simulink model "Q7_cartesian_space_solution"  (R2017a)
settings: Solver=FixedStepAuto  StartTime=0.0  StopTime=10  FixedStep=0.001  RelTol=0.00001
model workspace (MAT data in the model file):
  a_1 = 1
  a_2 = 1
  g = 9.8
  m_1 = 1
  m_2 = 1
  simulation_time = 4
  x1_0 = 1.9998
  x1_dot_0 = 0
  x1_dot_f = 0
  x1_double_dot_0 = 0
  x1_double_dot_f = 0
  x1_f = 0
  x2_0 = 0
  x2_dot_0 = 0
  x2_dot_f = 0
  x2_double_dot_0 = 0
  x2_double_dot_f = 0
  x2_f = 1
libraries: simulink x15
settings Model: Creator=Omer  LastModifiedBy=Omer
settings ModelReferenceCC: ModelReferenceMinAlgLoopOccurrences=on

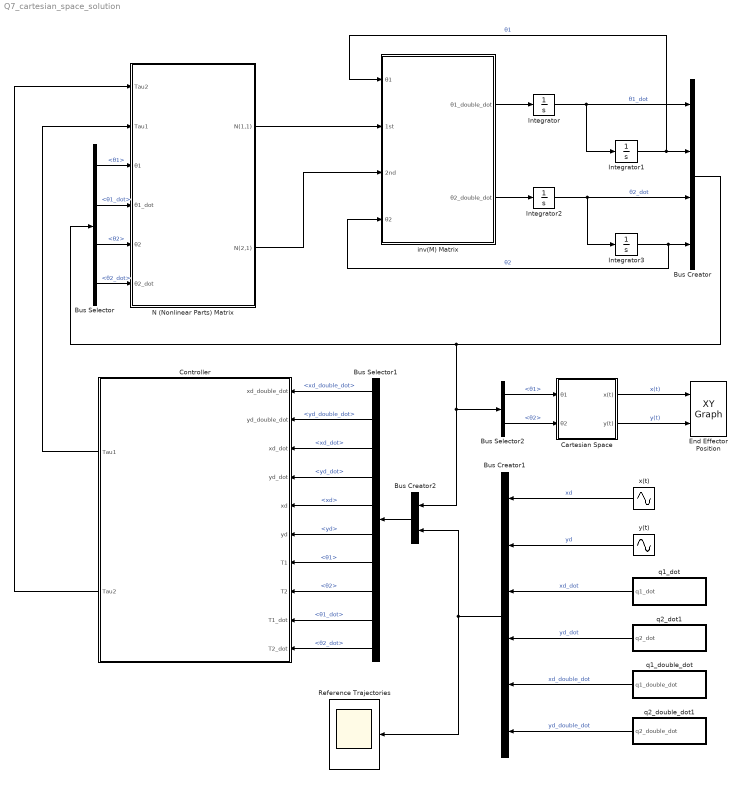
== system Q7_cartesian_space_solution ==
  Bus Creator : BusCreator  Inputs=4
  Bus Creator1 : BusCreator  Inputs=6
  Bus Creator2 : BusCreator  Inputs=2
  Bus Selector : BusSelector  OutputSignals=θ1,θ1_dot,θ2,θ2_dot
  Bus Selector1 : BusSelector  OutputSignals=signal2.xd_double_dot,signal2.yd_double_dot,signal2.xd_dot,signal2.yd_dot,signal2.xd,signal2.yd,signal1.θ1,signal1.θ2,signal1.θ1_dot,signal1.θ2_dot
  Bus Selector2 : BusSelector  OutputSignals=θ1,θ2
  "Cartesian Space " : Subsystem  TreatAsAtomicUnit=on
  Controller : MATLAB Function  TreatAsAtomicUnit=on
  End Effector Position : simulink/Sinks/XY Graph  xmin=-2  xmax=2  ymin=-1  ymax=2  st=-1
  Integrator : Integrator  UpperSaturationLimit=5  LowerSaturationLimit=-5
  Integrator1 : Integrator  InitialCondition=pi/6  UpperSaturationLimit=5  LowerSaturationLimit=-5
  Integrator2 : Integrator  UpperSaturationLimit=5  LowerSaturationLimit=-5
  Integrator3 : Integrator  InitialCondition=5*pi/6  UpperSaturationLimit=5  LowerSaturationLimit=-5
  N (Nonlinear Parts) Matrix : Subsystem  TreatAsAtomicUnit=on
  Reference Trajectories : Scope
  inv(M) Matrix : Subsystem  TreatAsAtomicUnit=on
  q1_dot : Subsystem  TreatAsAtomicUnit=on
  q1_double_dot : Subsystem  TreatAsAtomicUnit=on
  q2_dot1 : Subsystem  TreatAsAtomicUnit=on
  q2_double_dot1 : Subsystem  TreatAsAtomicUnit=on
  x(t) : Sin  Amplitude=0.5  Frequency=pi/5  SampleTime=0
  y(t) : Sin  Amplitude=0.5  Bias=1  Frequency=pi/5  Phase=-pi/2  SampleTime=0
  wires:
  N (Nonlinear Parts) Matrix/2(N(2,1)) -> inv(M) Matrix/3(2nd)
  N (Nonlinear Parts) Matrix/1(N(1,1)) -> inv(M) Matrix/2(1st)
  Bus Creator/1 -> Bus Selector2/1, Bus Creator2/1, Bus Selector/1
  inv(M) Matrix/2(θ2_double_dot) -> Integrator2/1
  Bus Selector/1 -> N (Nonlinear Parts) Matrix/3("θ1 ")  "<θ1>"
  Integrator2/1 -> Integrator3/1, Bus Creator/3  "θ2_dot"
  Integrator3/1 -> inv(M) Matrix/4(θ2), Bus Creator/4  "θ2"
  Integrator1/1 -> inv(M) Matrix/1(θ1), Bus Creator/2  "θ1"
  Bus Selector/3 -> N (Nonlinear Parts) Matrix/5(θ2)  "<θ2>"
  Bus Selector/2 -> N (Nonlinear Parts) Matrix/4(θ1_dot)  "<θ1_dot>"
  Integrator/1 -> Bus Creator/1, Integrator1/1  "θ1_dot"
  Bus Selector/4 -> N (Nonlinear Parts) Matrix/6(θ2_dot)  "<θ2_dot>"
  inv(M) Matrix/1(θ1_double_dot) -> Integrator/1
  Bus Selector2/1 -> "Cartesian Space "/1(θ1)  "<θ1>"
  Bus Selector2/2 -> "Cartesian Space "/2(θ2)  "<θ2>"
  "Cartesian Space "/1(x(t)) -> End Effector Position/1  "x(t)"
  "Cartesian Space "/2(y(t)) -> End Effector Position/2  "y(t)"
  Bus Creator2/1 -> Bus Selector1/1
  Bus Selector1/1 -> Controller/1(xd_double_dot)  "<xd_double_dot>"
  Bus Selector1/2 -> Controller/2(yd_double_dot)  "<yd_double_dot>"
  Bus Selector1/3 -> Controller/3(xd_dot)  "<xd_dot>"
  Bus Selector1/4 -> Controller/4(yd_dot)  "<yd_dot>"
  Bus Selector1/5 -> Controller/5(xd)  "<xd>"
  Bus Selector1/6 -> Controller/6(yd)  "<yd>"
  Bus Selector1/7 -> Controller/7(T1)  "<θ1>"
  Bus Selector1/8 -> Controller/8(T2)  "<θ2>"
  Bus Selector1/9 -> Controller/9(T1_dot)  "<θ1_dot>"
  Bus Selector1/10 -> Controller/10(T2_dot)  "<θ2_dot>"
  Controller/1(Tau1) -> N (Nonlinear Parts) Matrix/2(Tau1)
  Controller/2(Tau2) -> N (Nonlinear Parts) Matrix/1(Tau2)
  x(t)/1 -> Bus Creator1/1  "xd"
  q1_double_dot/1(q1_double_dot) -> Bus Creator1/5  "xd_double_dot"
  q2_dot1/1(q2_dot) -> Bus Creator1/4  "yd_dot"
  Bus Creator1/1 -> Reference Trajectories/1, Bus Creator2/2
  q2_double_dot1/1(q2_double_dot) -> Bus Creator1/6  "yd_double_dot"
  y(t)/1 -> Bus Creator1/2  "yd"
  q1_dot/1(q1_dot) -> Bus Creator1/3  "xd_dot"

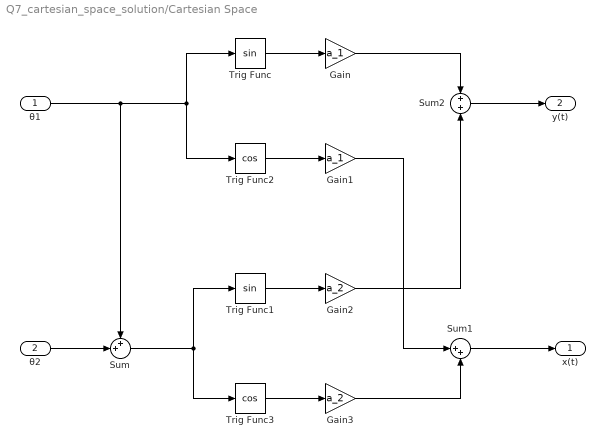
== system Q7_cartesian_space_solution/Cartesian Space  ==
  θ1 : Inport
  θ2 : Inport  Port=2
  Gain : Gain  Gain=a_1
  Gain1 : Gain  Gain=a_1
  Gain2 : Gain  Gain=a_2
  Gain3 : Gain  Gain=a_2
  Sum : Sum  Inputs=++|
  Sum1 : Sum  Inputs=|++
  Sum2 : Sum  Inputs=+|+
  Trig Func : Trigonometry
  Trig Func1 : Trigonometry
  Trig Func2 : Trigonometry  Operator=cos
  Trig Func3 : Trigonometry  Operator=cos
  x(t) : Outport
  y(t) : Outport  Port=2
  wires:
  θ1/1 -> Trig Func2/1, Trig Func/1, Sum/1
  θ2/1 -> Sum/2
  Sum/1 -> Trig Func3/1, Trig Func1/1
  Sum2/1 -> y(t)/1
  Sum1/1 -> x(t)/1
  Trig Func/1 -> Gain/1
  Gain/1 -> Sum2/1
  Trig Func2/1 -> Gain1/1
  Gain1/1 -> Sum1/1
  Trig Func1/1 -> Gain2/1
  Gain2/1 -> Sum2/2
  Trig Func3/1 -> Gain3/1
  Gain3/1 -> Sum1/2

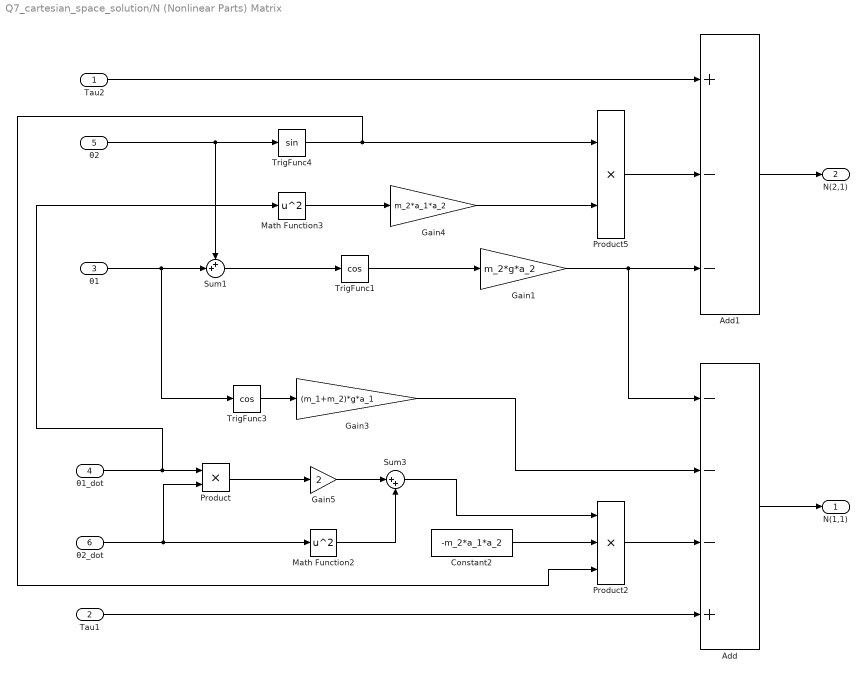
== system Q7_cartesian_space_solution/N (Nonlinear Parts) Matrix ==
  Tau2 : Inport
  Tau1 : Inport  Port=2
  "θ1 " : Inport  Port=3
  θ1_dot : Inport  Port=4
  θ2 : Inport  Port=5
  θ2_dot : Inport  Port=6
  Add : Sum  Inputs=---+
  Add1 : Sum  Inputs=+--
  Constant2 : Constant  Value=-m_2*a_1*a_2
  Gain1 : Gain  Gain=m_2*g*a_2
  Gain3 : Gain  Gain=(m_1+m_2)*g*a_1
  Gain4 : Gain  Gain=m_2*a_1*a_2
  Gain5 : Gain  Gain=2
  Math Function2 : Math  Operator=square  SaturateOnIntegerOverflow=on
  Math Function3 : Math  Operator=square  SaturateOnIntegerOverflow=on
  Product : Product
  Product2 : Product  Inputs=3
  Product5 : Product
  Sum1 : Sum  Inputs=++|
  Sum3 : Sum  Inputs=|++
  TrigFunc1 : Trigonometry  Operator=cos
  TrigFunc3 : Trigonometry  Operator=cos
  TrigFunc4 : Trigonometry
  N(1,1) : Outport
  N(2,1) : Outport  Port=2
  wires:
  Product2/1 -> Add/3
  Gain3/1 -> Add/2
  θ2/1 -> TrigFunc4/1, Sum1/1
  TrigFunc4/1 -> Product2/3, Product5/1
  Add1/1 -> N(2,1)/1
  Math Function3/1 -> Gain4/1
  θ1_dot/1 -> Product/1, Math Function3/1
  θ2_dot/1 -> Product/2, Math Function2/1
  Sum1/1 -> TrigFunc1/1
  Add/1 -> N(1,1)/1
  Sum3/1 -> Product2/1
  Math Function2/1 -> Sum3/2
  Tau2/1 -> Add1/1
  Constant2/1 -> Product2/2
  TrigFunc3/1 -> Gain3/1
  TrigFunc1/1 -> Gain1/1
  "θ1 "/1 -> TrigFunc3/1, Sum1/2
  Product5/1 -> Add1/2
  Tau1/1 -> Add/4
  Gain4/1 -> Product5/2
  Gain1/1 -> Add1/3, Add/1
  Product/1 -> Gain5/1
  Gain5/1 -> Sum3/1

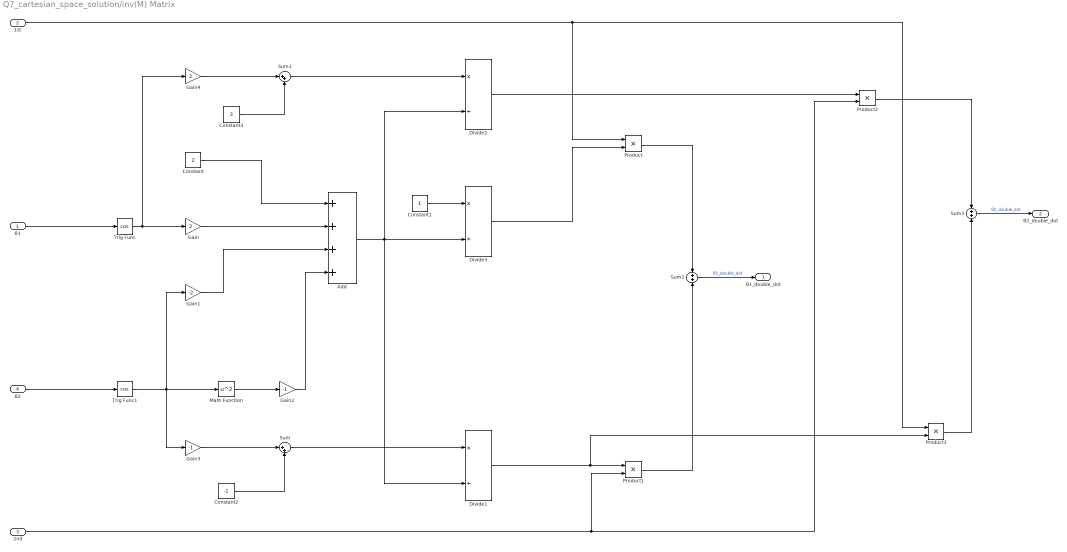
== system Q7_cartesian_space_solution/inv(M) Matrix ==
  θ1 : Inport
  1st : Inport  Port=2
  2nd : Inport  Port=3
  θ2 : Inport  Port=4
  Add : Sum  Inputs=4
  Constant : Constant  Value=2
  Constant1 : Constant
  Constant2 : Constant  Value=-1
  Constant3 : Constant  Value=3
  Divide1 : Product  Inputs=*/
  Divide2 : Product  Inputs=*/
  Divide3 : Product  Inputs=*/
  Gain : Gain  Gain=2
  Gain1 : Gain  Gain=-2
  Gain2 : Gain  Gain=-1
  Gain3 : Gain  Gain=-1
  Gain4 : Gain  Gain=2
  Math Function : Math  Operator=square  SaturateOnIntegerOverflow=on
  Product{,1..3} (4 alike) : Product
  Sum : Sum  Inputs=|++
  Sum1 : Sum  Inputs=|++
  Sum2 : Sum  Inputs=+|+
  Sum3 : Sum  Inputs=+|+
  Trig Func : Trigonometry  Operator=cos
  Trig Func1 : Trigonometry  Operator=cos
  θ1_double_dot : Outport
  θ2_double_dot : Outport  Port=2
  wires:
  Add/1 -> Divide2/2, Divide3/2, Divide1/2
  θ1/1 -> Trig Func/1
  θ2/1 -> Trig Func1/1
  Trig Func1/1 -> Gain3/1, Gain1/1, Math Function/1
  Trig Func/1 -> Gain4/1, Gain/1
  Constant/1 -> Add/1
  Gain/1 -> Add/2
  Gain1/1 -> Add/3
  Constant1/1 -> Divide3/1
  Math Function/1 -> Gain2/1
  Gain2/1 -> Add/4
  Gain3/1 -> Sum/1
  Constant2/1 -> Sum/2
  Sum/1 -> Divide1/1
  Constant3/1 -> Sum1/2
  Gain4/1 -> Sum1/1
  1st/1 -> Product/1, Product3/1
  Divide3/1 -> Product/2
  Divide1/1 -> Product3/2, Product1/1
  2nd/1 -> Product2/2, Product1/2
  Product/1 -> Sum2/1
  Product1/1 -> Sum2/2
  Sum2/1 -> θ1_double_dot/1  "θ1_double_dot"
  Sum1/1 -> Divide2/1
  Divide2/1 -> Product2/1
  Product2/1 -> Sum3/1
  Sum3/1 -> θ2_double_dot/1  "θ2_double_dot"
  Product3/1 -> Sum3/2

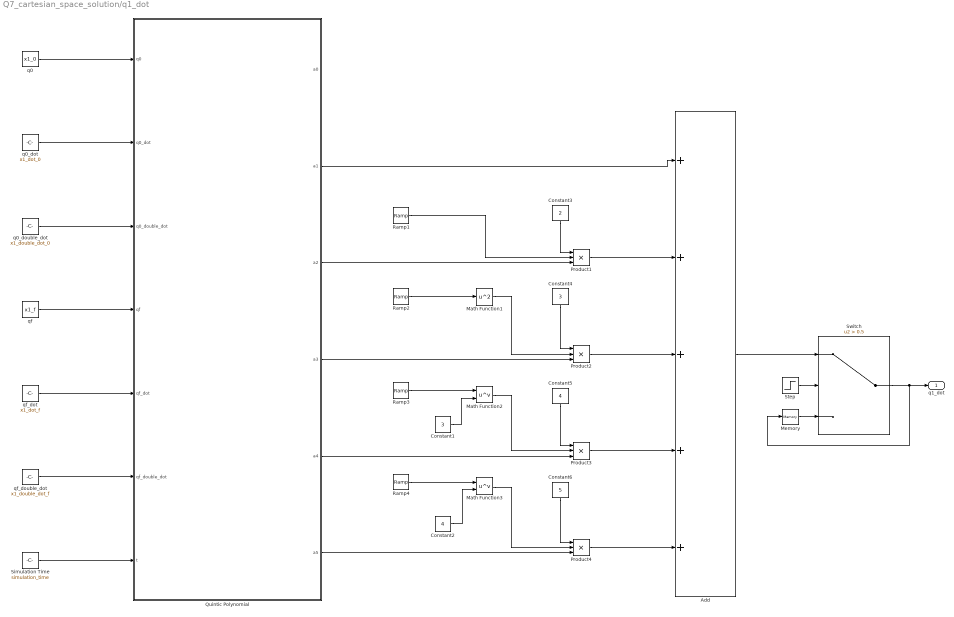
== system Q7_cartesian_space_solution/q1_dot ==
  Add : Sum  Inputs=5
  Constant1 : Constant  Value=3
  Constant2 : Constant  Value=4
  Constant3 : Constant  Value=2
  Constant4 : Constant  Value=3
  Constant5 : Constant  Value=4
  Constant6 : Constant  Value=5
  Math Function1 : Math  Operator=square  SaturateOnIntegerOverflow=on
  Math Function2 : Math  Operator=pow  SaturateOnIntegerOverflow=on
  Math Function3 : Math  Operator=pow  SaturateOnIntegerOverflow=on
  Memory : Memory
  Product{1..4} (4 alike) : Product  Inputs=3
  Quintic Polynomial : MATLAB Function  TreatAsAtomicUnit=on
  Ramp{1..4} (4 alike) : simulink/Sources/Ramp  slope=1  start=0  X0=0
  Simulation Time : Constant  Value=simulation_time
  Step : Step  Time=simulation_time  Before=1  After=0  SampleTime=0
  Switch : Switch  Criteria=u2 > Threshold  Threshold=0.5
  q0 : Constant  Value=x1_0
  q0_dot : Constant  Value=x1_dot_0
  q0_double_dot : Constant  Value=x1_double_dot_0
  qf : Constant  Value=x1_f
  qf_dot : Constant  Value=x1_dot_f
  qf_double_dot : Constant  Value=x1_double_dot_f
  q1_dot : Outport
  wires:
  Constant6/1 -> Product4/1
  Ramp1/1 -> Product1/2
  Ramp3/1 -> Math Function2/1
  Product1/1 -> Add/2
  Math Function1/1 -> Product2/2
  Simulation Time/1 -> Quintic Polynomial/7(t)
  Ramp4/1 -> Math Function3/1
  qf_double_dot/1 -> Quintic Polynomial/6(qf_double_dot)
  Quintic Polynomial/6(a5) -> Product4/3
  q0_double_dot/1 -> Quintic Polynomial/3(q0_double_dot)
  Product2/1 -> Add/3
  Quintic Polynomial/4(a3) -> Product2/3
  q0_dot/1 -> Quintic Polynomial/2(q0_dot)
  q0/1 -> Quintic Polynomial/1(q0)
  Quintic Polynomial/2(a1) -> Add/1
  Ramp2/1 -> Math Function1/1
  Math Function2/1 -> Product3/2
  Constant5/1 -> Product3/1
  Constant4/1 -> Product2/1
  Product3/1 -> Add/4
  Math Function3/1 -> Product4/2
  qf_dot/1 -> Quintic Polynomial/5(qf_dot)
  Constant3/1 -> Product1/1
  Constant1/1 -> Math Function2/2
  Constant2/1 -> Math Function3/2
  Product4/1 -> Add/5
  Quintic Polynomial/5(a4) -> Product3/3
  qf/1 -> Quintic Polynomial/4(qf)
  Quintic Polynomial/3(a2) -> Product1/3
  Memory/1 -> Switch/3
  Add/1 -> Switch/1
  Switch/1 -> q1_dot/1, Memory/1
  Step/1 -> Switch/2

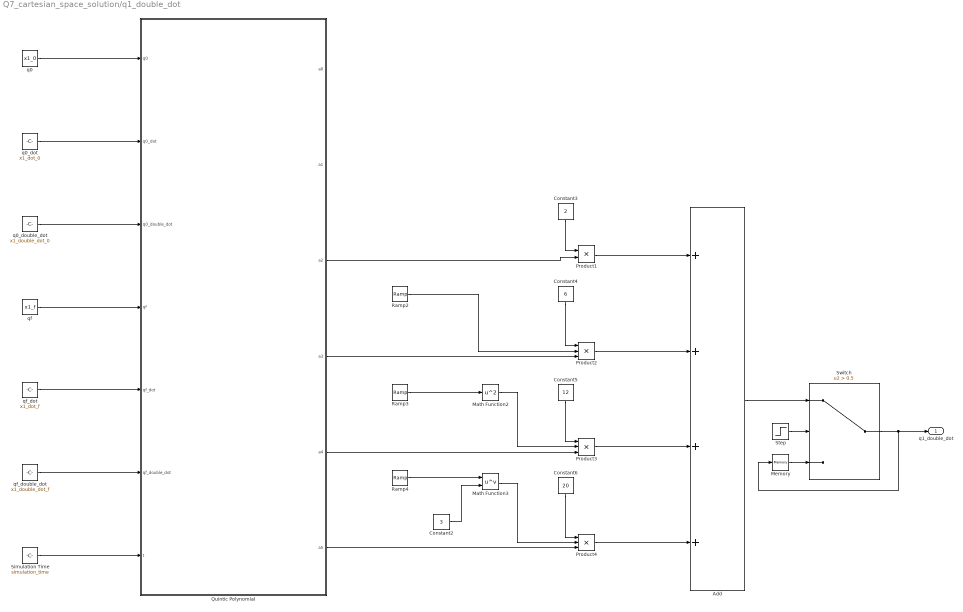
== system Q7_cartesian_space_solution/q1_double_dot ==
  Add : Sum  Inputs=4
  Constant2 : Constant  Value=3
  Constant3 : Constant  Value=2
  Constant4 : Constant  Value=6
  Constant5 : Constant  Value=12
  Constant6 : Constant  Value=20
  Math Function2 : Math  Operator=square  SaturateOnIntegerOverflow=on
  Math Function3 : Math  Operator=pow  SaturateOnIntegerOverflow=on
  Memory : Memory
  Product1 : Product
  Product2 : Product  Inputs=3
  Product3 : Product  Inputs=3
  Product4 : Product  Inputs=3
  Quintic Polynomial : MATLAB Function  TreatAsAtomicUnit=on
  Ramp2 : simulink/Sources/Ramp  slope=1  start=0  X0=0
  Ramp3 : simulink/Sources/Ramp  slope=1  start=0  X0=0
  Ramp4 : simulink/Sources/Ramp  slope=1  start=0  X0=0
  Simulation Time : Constant  Value=simulation_time
  Step : Step  Time=simulation_time  Before=1  After=0  SampleTime=0
  Switch : Switch  Criteria=u2 > Threshold  Threshold=0.5
  q0 : Constant  Value=x1_0
  q0_dot : Constant  Value=x1_dot_0
  q0_double_dot : Constant  Value=x1_double_dot_0
  qf : Constant  Value=x1_f
  qf_dot : Constant  Value=x1_dot_f
  qf_double_dot : Constant  Value=x1_double_dot_f
  q1_double_dot : Outport
  wires:
  Quintic Polynomial/6(a5) -> Product4/3
  Quintic Polynomial/5(a4) -> Product3/3
  Quintic Polynomial/4(a3) -> Product2/3
  Quintic Polynomial/3(a2) -> Product1/2
  q0_dot/1 -> Quintic Polynomial/2(q0_dot)
  Constant4/1 -> Product2/1
  Constant5/1 -> Product3/1
  Constant6/1 -> Product4/1
  Math Function3/1 -> Product4/2
  Product1/1 -> Add/1
  Constant3/1 -> Product1/1
  Math Function2/1 -> Product3/2
  Product2/1 -> Add/2
  Ramp2/1 -> Product2/2
  Ramp4/1 -> Math Function3/1
  Product3/1 -> Add/3
  qf/1 -> Quintic Polynomial/4(qf)
  qf_dot/1 -> Quintic Polynomial/5(qf_dot)
  Product4/1 -> Add/4
  q0/1 -> Quintic Polynomial/1(q0)
  Constant2/1 -> Math Function3/2
  q0_double_dot/1 -> Quintic Polynomial/3(q0_double_dot)
  Ramp3/1 -> Math Function2/1
  qf_double_dot/1 -> Quintic Polynomial/6(qf_double_dot)
  Simulation Time/1 -> Quintic Polynomial/7(t)
  Memory/1 -> Switch/3
  Add/1 -> Switch/1
  Switch/1 -> q1_double_dot/1, Memory/1
  Step/1 -> Switch/2

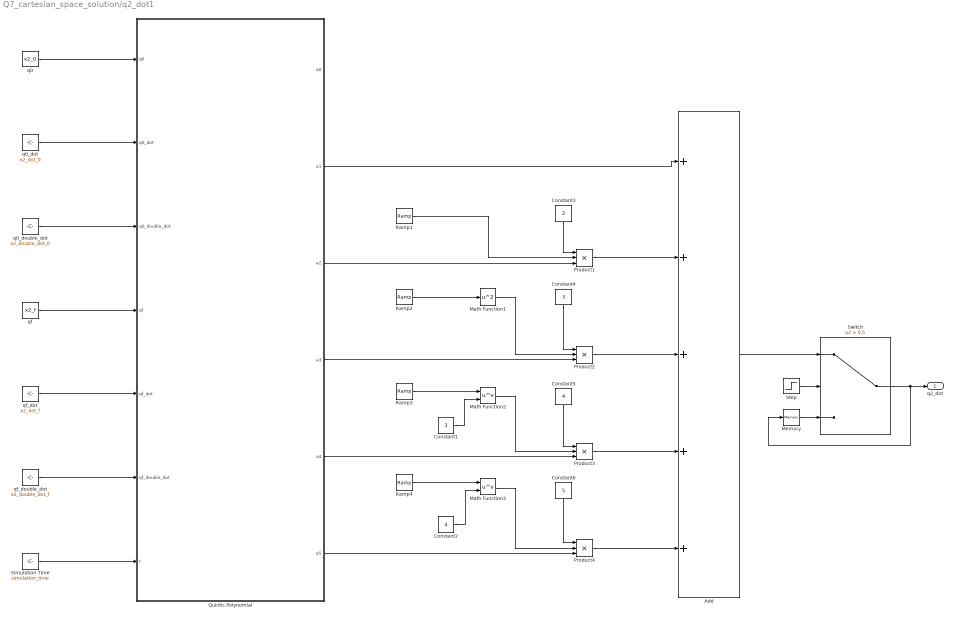
== system Q7_cartesian_space_solution/q2_dot1 ==
  Add : Sum  Inputs=5
  Constant1 : Constant  Value=3
  Constant2 : Constant  Value=4
  Constant3 : Constant  Value=2
  Constant4 : Constant  Value=3
  Constant5 : Constant  Value=4
  Constant6 : Constant  Value=5
  Math Function1 : Math  Operator=square  SaturateOnIntegerOverflow=on
  Math Function2 : Math  Operator=pow  SaturateOnIntegerOverflow=on
  Math Function3 : Math  Operator=pow  SaturateOnIntegerOverflow=on
  Memory : Memory
  Product{1..4} (4 alike) : Product  Inputs=3
  Quintic Polynomial : MATLAB Function  TreatAsAtomicUnit=on
  Ramp{1..4} (4 alike) : simulink/Sources/Ramp  slope=1  start=0  X0=0
  Simulation Time : Constant  Value=simulation_time
  Step : Step  Time=simulation_time  Before=1  After=0  SampleTime=0
  Switch : Switch  Criteria=u2 > Threshold  Threshold=0.5
  q0 : Constant  Value=x2_0
  q0_dot : Constant  Value=x2_dot_0
  q0_double_dot : Constant  Value=x2_double_dot_0
  qf : Constant  Value=x2_f
  qf_dot : Constant  Value=x2_dot_f
  qf_double_dot : Constant  Value=x2_double_dot_f
  q2_dot : Outport
  wires:
  Quintic Polynomial/2(a1) -> Add/1
  Product1/1 -> Add/2
  Product2/1 -> Add/3
  Product3/1 -> Add/4
  Product4/1 -> Add/5
  Ramp1/1 -> Product1/2
  Ramp2/1 -> Math Function1/1
  Ramp3/1 -> Math Function2/1
  Ramp4/1 -> Math Function3/1
  Quintic Polynomial/3(a2) -> Product1/3
  Math Function1/1 -> Product2/2
  Math Function2/1 -> Product3/2
  Math Function3/1 -> Product4/2
  Quintic Polynomial/4(a3) -> Product2/3
  Quintic Polynomial/5(a4) -> Product3/3
  Quintic Polynomial/6(a5) -> Product4/3
  Constant1/1 -> Math Function2/2
  Constant2/1 -> Math Function3/2
  q0/1 -> Quintic Polynomial/1(q0)
  q0_dot/1 -> Quintic Polynomial/2(q0_dot)
  q0_double_dot/1 -> Quintic Polynomial/3(q0_double_dot)
  qf/1 -> Quintic Polynomial/4(qf)
  qf_dot/1 -> Quintic Polynomial/5(qf_dot)
  qf_double_dot/1 -> Quintic Polynomial/6(qf_double_dot)
  Simulation Time/1 -> Quintic Polynomial/7(t)
  Constant3/1 -> Product1/1
  Constant4/1 -> Product2/1
  Constant5/1 -> Product3/1
  Constant6/1 -> Product4/1
  Memory/1 -> Switch/3
  Add/1 -> Switch/1
  Switch/1 -> q2_dot/1, Memory/1
  Step/1 -> Switch/2

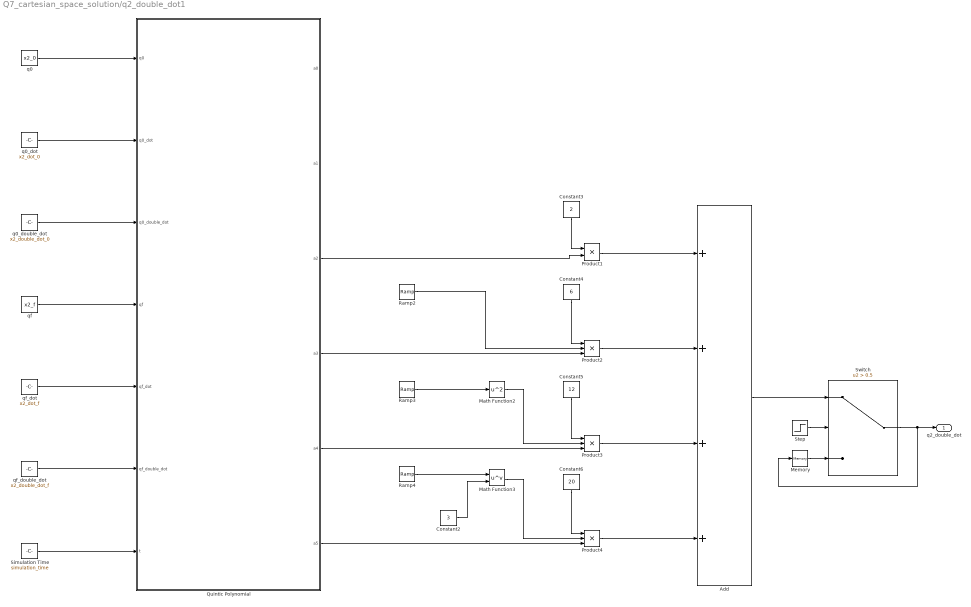
== system Q7_cartesian_space_solution/q2_double_dot1 ==
  Add : Sum  Inputs=4
  Constant2 : Constant  Value=3
  Constant3 : Constant  Value=2
  Constant4 : Constant  Value=6
  Constant5 : Constant  Value=12
  Constant6 : Constant  Value=20
  Math Function2 : Math  Operator=square  SaturateOnIntegerOverflow=on
  Math Function3 : Math  Operator=pow  SaturateOnIntegerOverflow=on
  Memory : Memory
  Product1 : Product
  Product2 : Product  Inputs=3
  Product3 : Product  Inputs=3
  Product4 : Product  Inputs=3
  Quintic Polynomial : MATLAB Function  TreatAsAtomicUnit=on
  Ramp2 : simulink/Sources/Ramp  slope=1  start=0  X0=0
  Ramp3 : simulink/Sources/Ramp  slope=1  start=0  X0=0
  Ramp4 : simulink/Sources/Ramp  slope=1  start=0  X0=0
  Simulation Time : Constant  Value=simulation_time
  Step : Step  Time=simulation_time  Before=1  After=0  SampleTime=0
  Switch : Switch  Criteria=u2 > Threshold  Threshold=0.5
  q0 : Constant  Value=x2_0
  q0_dot : Constant  Value=x2_dot_0
  q0_double_dot : Constant  Value=x2_double_dot_0
  qf : Constant  Value=x2_f
  qf_dot : Constant  Value=x2_dot_f
  qf_double_dot : Constant  Value=x2_double_dot_f
  q2_double_dot : Outport
  wires:
  Product1/1 -> Add/1
  Product2/1 -> Add/2
  Product3/1 -> Add/3
  Product4/1 -> Add/4
  Ramp3/1 -> Math Function2/1
  Ramp4/1 -> Math Function3/1
  Quintic Polynomial/3(a2) -> Product1/2
  Ramp2/1 -> Product2/2
  Math Function2/1 -> Product3/2
  Math Function3/1 -> Product4/2
  Quintic Polynomial/4(a3) -> Product2/3
  Quintic Polynomial/5(a4) -> Product3/3
  Quintic Polynomial/6(a5) -> Product4/3
  Constant2/1 -> Math Function3/2
  q0/1 -> Quintic Polynomial/1(q0)
  q0_dot/1 -> Quintic Polynomial/2(q0_dot)
  q0_double_dot/1 -> Quintic Polynomial/3(q0_double_dot)
  qf/1 -> Quintic Polynomial/4(qf)
  qf_dot/1 -> Quintic Polynomial/5(qf_dot)
  qf_double_dot/1 -> Quintic Polynomial/6(qf_double_dot)
  Simulation Time/1 -> Quintic Polynomial/7(t)
  Constant3/1 -> Product1/1
  Constant4/1 -> Product2/1
  Constant5/1 -> Product3/1
  Constant6/1 -> Product4/1
  Memory/1 -> Switch/3
  Add/1 -> Switch/1
  Switch/1 -> q2_double_dot/1, Memory/1
  Step/1 -> Switch/2

== matlab function Q7_cartesian_space_solution/Controller ==
  data: xd_double_dot input; yd_double_dot input; xd_dot input; yd_dot input; xd input; yd input; Tau1 output; T1 input; T2 input; T1_dot input; T2_dot input; Tau2 output
function [Tau1, Tau2] = fcn(xd_double_dot, yd_double_dot, xd_dot, yd_dot, xd, yd, T1, T2, T1_dot, T2_dot)
Kp = 10000; Kv = 2*sqrt(Kp); g = 9.8;  
Xd_double_dot = [xd_double_dot; yd_double_dot];

J = @(T1,T2) [-sin(T1)-sin(T1+T2), -sin(T1+T2); cos(T1)+cos(T1+T2), cos(T1+T2)];
Jdot = @(T1,T2) [-cos(T1)*T1_dot-cos(T1+T2)*(T1_dot+T2_dot), -cos(T1+T2)*(T1_dot+T2_dot);
        -sin(T1)*T1_dot-sin(T1+T2)*(T1_dot+T2_dot), -sin(T1+T2)*(T1_dot+T2_dot)];
Jinv = @(T1,T2) inv(J(T1,T2));
JTrnsp = @(T1,T2) (J(T1,T2))';
JinvTrnsp = @(T1,T2) (Jinv(T1,T2))';

X = [cos(T1+T2)+cos(T1); sin(T1+T2)+sin(T1)];
e = [xd - X(1,1); yd - X(2,1)];
X_dot = J(T1,T2)*[T1_dot; T2_dot];
e_dot = [xd_dot - X_dot(1,1); yd_dot - X_dot(2,1)];

M = @(T2) [3+2*cos(T2) 1+cos(T2); 1+cos(T2) 1];
N = @(T1,T2,T1_dot,T2_dot) [-(2*T1_dot*T2_dot+T2_dot^2)*sin(T2) + 2*g*cos(T1) + g*cos(T1+T2);
     T1_dot^2*sin(T2) + g*cos(T1+T2)];

Mx = @(T1,T2) JinvTrnsp(T1,T2)*M(T2)*Jinv(T1,T2);
Nx = @(T1,T2,T1_dot,T2_dot) JinvTrnsp(T1,T2) ...
    *(N(T1,T2,T1_dot,T2_dot) - M(T2)*Jinv(T1,T2)*Jdot(T1,T2)*[T1_dot; T2_dot]);

F = Mx(T1,T2)*(Xd_double_dot + [Kv 0; 0 Kv]*e_dot + [Kp 0; 0 Kp]*e) + Nx(T1,T2,T1_dot,T2_dot);
Tau = JTrnsp(T1,T2)*F;
Tau1 = Tau(1,1);
Tau2 = Tau(2,1);

== matlab function Q7_cartesian_space_solution/q1_dot/Quintic Polynomial ==
  data: q0 input; a0 output; a1 output; a2 output; a3 output; a4 output; a5 output; q0_dot input; q0_double_dot input; qf input; qf_dot input; qf_double_dot input; t input
function [a0, a1, a2, a3, a4, a5] = fcn(q0, q0_dot, q0_double_dot, qf, qf_dot, qf_double_dot, t)

T = [1 0 0 0 0 0;
     0 1 0 0 0 0;
     0 0 2 0 0 0;
     1 t t^2 t^3 t^4 t^5;
     0 1 2*t 3*t^2 4*t^3 5*t^4;
     0 0 2 6*t 12*t^2 20*t^3];

q = [q0, q0_dot, q0_double_dot, qf, qf_dot, qf_double_dot]';
Q = inv(T)*q;
a0=Q(1); a1=Q(2); a2=Q(3); a3=Q(4); a4=Q(5); a5=Q(6);

== matlab function Q7_cartesian_space_solution/q1_double_dot/Quintic Polynomial ==
  data: q0 input; a0 output; a1 output; a2 output; a3 output; a4 output; a5 output; q0_dot input; q0_double_dot input; qf input; qf_dot input; qf_double_dot input; t input
function [a0, a1, a2, a3, a4, a5] = fcn(q0, q0_dot, q0_double_dot, qf, qf_dot, qf_double_dot, t)

T = [1 0 0 0 0 0;
     0 1 0 0 0 0;
     0 0 2 0 0 0;
     1 t t^2 t^3 t^4 t^5;
     0 1 2*t 3*t^2 4*t^3 5*t^4;
     0 0 2 6*t 12*t^2 20*t^3];

q = [q0, q0_dot, q0_double_dot, qf, qf_dot, qf_double_dot]';
Q = inv(T)*q;
a0=Q(1); a1=Q(2); a2=Q(3); a3=Q(4); a4=Q(5); a5=Q(6);

== matlab function Q7_cartesian_space_solution/q2_dot1/Quintic Polynomial ==
  data: q0 input; a0 output; a1 output; a2 output; a3 output; a4 output; a5 output; q0_dot input; q0_double_dot input; qf input; qf_dot input; qf_double_dot input; t input
function [a0, a1, a2, a3, a4, a5] = fcn(q0, q0_dot, q0_double_dot, qf, qf_dot, qf_double_dot, t)

T = [1 0 0 0 0 0;
     0 1 0 0 0 0;
     0 0 2 0 0 0;
     1 t t^2 t^3 t^4 t^5;
     0 1 2*t 3*t^2 4*t^3 5*t^4;
     0 0 2 6*t 12*t^2 20*t^3];

q = [q0, q0_dot, q0_double_dot, qf, qf_dot, qf_double_dot]';
Q = inv(T)*q;
a0=Q(1); a1=Q(2); a2=Q(3); a3=Q(4); a4=Q(5); a5=Q(6);

== matlab function Q7_cartesian_space_solution/q2_double_dot1/Quintic Polynomial ==
  data: q0 input; a0 output; a1 output; a2 output; a3 output; a4 output; a5 output; q0_dot input; q0_double_dot input; qf input; qf_dot input; qf_double_dot input; t input
function [a0, a1, a2, a3, a4, a5] = fcn(q0, q0_dot, q0_double_dot, qf, qf_dot, qf_double_dot, t)

T = [1 0 0 0 0 0;
     0 1 0 0 0 0;
     0 0 2 0 0 0;
     1 t t^2 t^3 t^4 t^5;
     0 1 2*t 3*t^2 4*t^3 5*t^4;
     0 0 2 6*t 12*t^2 20*t^3];

q = [q0, q0_dot, q0_double_dot, qf, qf_dot, qf_double_dot]';
Q = inv(T)*q;
a0=Q(1); a1=Q(2); a2=Q(3); a3=Q(4); a4=Q(5); a5=Q(6);
